simulink model "untitled"  (R2015a)
settings: Solver=ode45  StartTime=0.0  StopTime=10.0  RelTol=1e-3
settings Model: Creator=Fer  LastModifiedBy=Fer

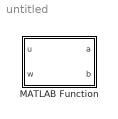
== system untitled ==
  MATLAB Function : MATLAB Function  TreatAsAtomicUnit=on

== matlab function untitled/MATLAB Function ==
  data: u input; a output; w input; b output
function [a,b] = fcn(u,w)
%#codegen
a=1
b=1
y = u;
